simulink model "ME565_Simulation2_QuarterCar_NonLinearF"  (R2025b)
settings: Solver=VariableStepAuto  StartTime=0.0  StopTime=10.0  RelTol=1e-3
values from neighbouring files (symbols this model uses):
  Ks = 100    [quarter_car_simulation.m]
  Kt = 1000    [quarter_car_simulation.m]
  ms = Ws/g    (= 2.59067357513)    [quarter_car_simulation.m]
  mu = Wu/g    (= 0.259067357513)    [quarter_car_simulation.m]

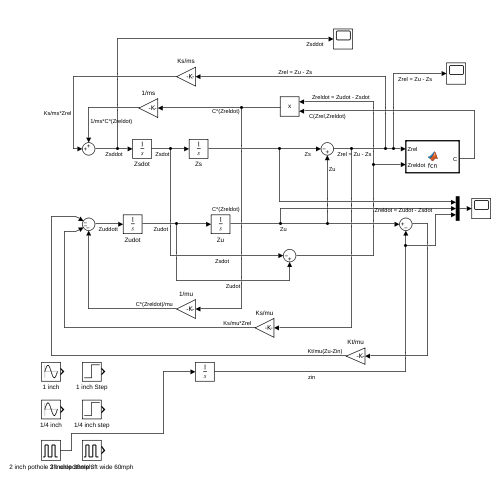
[thumbnail: Simulink's stored preview of the top-level diagram]
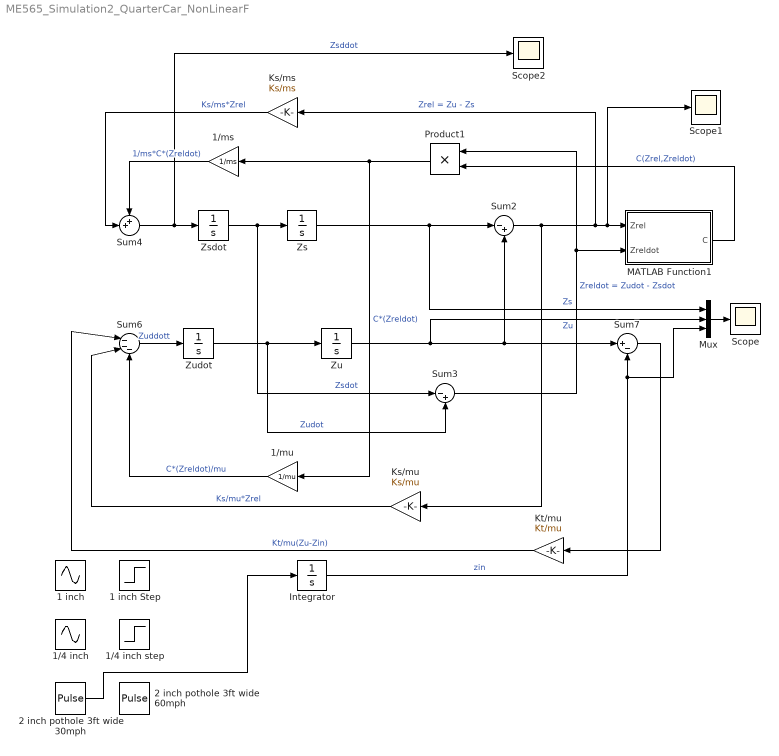
== system ME565_Simulation2_QuarterCar_NonLinearF ==
  1 inch : Sin  Frequency=2*pi*1  SampleTime=0
  1 inch Step : Step  Time=2  SampleTime=0
  1/4 inch : Sin  Amplitude=0.25  Frequency=2*pi*10  SampleTime=0
  1/4 inch step : Step  Time=2  After=0.25  SampleTime=0
  1/ms : Gain  Gain=1/ms
  1/mu : Gain  Gain=1/mu
  2 inch pothole 3ft wide 30mph : DiscretePulseGenerator  PulseType=Time based  Amplitude=-2  Period=5  PulseWidth=(0.068/5)*100  PhaseDelay=2
  2 inch pothole 3ft wide 60mph : DiscretePulseGenerator  PulseType=Time based  Amplitude=-2  Period=5  PulseWidth=(0.0345/5)*100  PhaseDelay=2
  Integrator : Integrator
  Ks/ms : Gain  Gain=Ks/ms
  Ks/mu : Gain  Gain=Ks/mu
  Kt/mu : Gain  Gain=Kt/mu
  MATLAB Function1 : MATLAB Function  TreatAsAtomicUnit=on
  Mux : Mux  Inputs=3
  Product1 : Product
  Scope : Scope
      settings: ActiveDisplayYMinimum=-0.41355598465512489  ActiveDisplayYMaximum=0.045950664961680536
  Scope1 : Scope
      settings: ActiveDisplayYMinimum=-0.087130325766950692  ActiveDisplayYMaximum=0.10562964168131443
  Scope2 : Scope
      settings: ActiveDisplayYMinimum=-26.817230497788383  ActiveDisplayYMaximum=13.374289341406987  DataLoggingVariableName=ScopeData2
  Sum2 : Sum  Inputs=|-+
  Sum3 : Sum  Inputs=|-+
  Sum4 : Sum  Inputs=++|
  Sum6 : Sum  Inputs=|---
  Sum7 : Sum  Inputs=|+-
  Zs : Integrator
  Zsdot : Integrator
  Zu : Integrator
  Zudot : Integrator
  wires:
  Zsdot/1 -> Zs/1, Sum3/1  "Zsdot"
  Zudot/1 -> Sum3/2, Zu/1  "Zudot"
  Zs/1 -> Mux/1, Sum2/1  "Zs"
  Zu/1 -> Sum7/1, Sum2/2, Mux/2  "Zu"
  Integrator/1 -> Mux/3, Sum7/2  "zin"
  Sum3/1 -> Product1/1, MATLAB Function1/2(Zreldot)  "Zreldot = Zudot - Zsdot"
  Sum4/1 -> Scope2/1, Zsdot/1  "Zsddot"
  Sum7/1 -> Kt/mu/1
  Sum2/1 -> Ks/mu/1, Ks/ms/1, Scope1/1, MATLAB Function1/1(Zrel)  "Zrel = Zu - Zs"
  MATLAB Function1/1(C) -> Product1/2  "C(Zrel,Zreldot)"
  Product1/1 -> 1/mu/1, 1/ms/1  "C*(Zreldot)"
  1/ms/1 -> Sum4/1  "1/ms*C*(Zreldot)"
  Ks/ms/1 -> Sum4/2  "Ks/ms*Zrel"
  Ks/mu/1 -> Sum6/2  "Ks/mu*Zrel"
  Kt/mu/1 -> Sum6/1  "Kt/mu(Zu-Zin)"
  1/mu/1 -> Sum6/3  "C*(Zreldot)/mu"
  Sum6/1 -> Zudot/1  "Zuddott"
  Mux/1 -> Scope/1
  2 inch pothole 3ft wide 30mph/1 -> Integrator/1

== matlab function ME565_Simulation2_QuarterCar_NonLinearF/MATLAB Function1 ==
  data: Zrel input; C output; Zreldot input
function C = fcn(Zrel, Zreldot)

%%%%%%%%

Cc = 20;
Cr = 50;
k = 5;

%%%%%

if Zreldot > 0

    C_base = Cc;

else
   
    C_base = Cr;

end

%%%%%%Progressive Stroke Effect

C = C_base + k*abs(Zrel);

end
